simulink model "slproject_f14"  (R2023a)
settings: Solver=VariableStepAuto  StartTime=0.0  StopTime=5  MaxStep=0.1  RelTol=1e-3  EnableMultiTasking=on
undefined symbols (not defined in the file): g, Uo
libraries: wind_gust_lib x1
settings Model: DataDictionary=system_model.sldd  EnableAccessToBaseWorkspace=off  ModifiedByFormat=The MathWorks Inc.  Creator=The MathWorks, Inc.  LastModifiedBy=The MathWorks Inc.
settings SolverCC: AlgebraicLoopSolver=TrustRegion
settings DataIOCC: LimitDataPoints=on  SaveFormat=Array  SaveOutput=off  SignalLogging=off  SaveTime=off  ReturnWorkspaceOutputs=off  SignalLoggingName=slproject_f14
settings OptimizationCC: ExpressionDepthLimit=2147483647  InitFltsAndDblsToZero=on  LifeSpan=inf
settings DebuggingCC: SaveWithParameterizedLinksMsg=none  UnderspecifiedInitializationDetection=Classic  MergeDetectMultiDrivingBlocksExec=none  SignalResolutionControl=TryResolveAllWithWarning  SolverPrmCheckMsg=warning  MultiTaskDSMMsg=warning  MultiTaskCondExecSysMsg=none  FcnCallInpInsideContextMsg=warning  UnconnectedInputMsg=warning  UnconnectedOutputMsg=warning  UnconnectedLineMsg=warning  AllowSymbolicDim=off  StateNameClashWarn=warning  SFUnexpectedBacktrackingDiag=warning  SFNoUnconditionalDefaultTransitionDiag=warning  SFExecutionAtInitializationDiag=none  ArithmeticOperatorsInVariantConditions=warning
settings HardwareCC: ProdBitPerPointer=32  ProdLargestAtomicFloat=None  ProdIntDivRoundTo=Undefined  ProdEndianess=Unspecified  ProdWordSize=32  ProdHWDeviceType=32-bit Generic
settings ModelReferenceCC: EnableRefExpFcnMdlSchedulingChecks=on  ModelReferenceMinAlgLoopOccurrences=on  PropagateSignalLabelsOutOfModel=off
settings SFSimCC: SimUseLocalCustomCode=off  CustomCodeUndefinedFunction=UseInterfaceOnly
settings RTWCC: RTWUseLocalCustomCode=off
settings CodeAppCC: StateflowObjectComments=on
settings GRTTargetCC: TargetFcnLib=ansi_tfl_tmw.mat  TargetLangStandard=C89/C90 (ANSI)  CombineOutputUpdateFcns=off  GRTInterface=on
settings ConfigComp: CovMetricSettings=dw  CovSaveCumulativeToWorkspaceVar=on  CovSaveSingleToWorkspaceVar=on  CovExternalEMLEnable=off  CovSFcnEnable=off

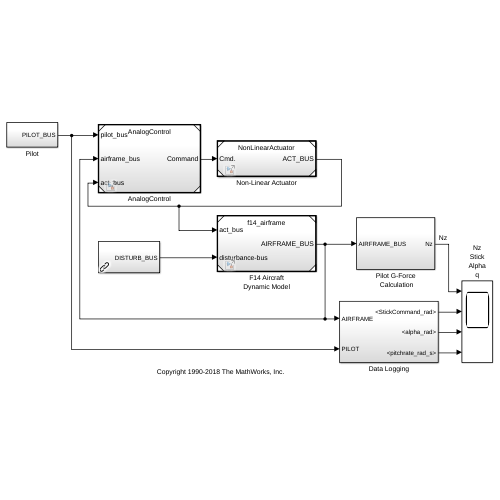
[thumbnail: Simulink's stored preview of the top-level diagram]
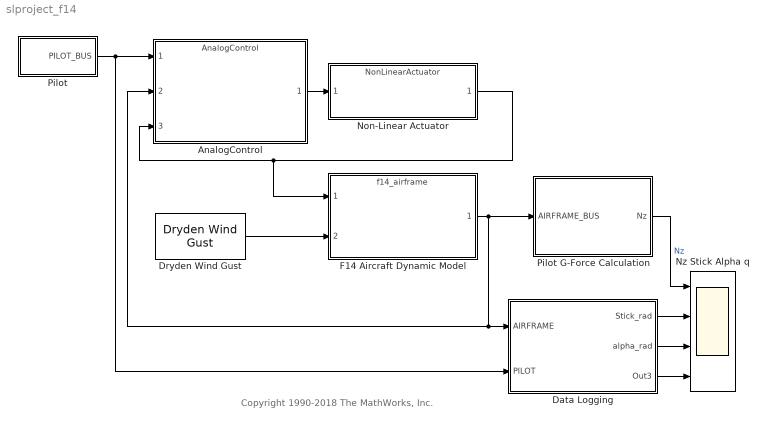
== system slproject_f14 ==
  note: Copyright 1990-2018 The MathWorks, Inc.
  AnalogControl : ModelReference  ModelNameDialog=AnalogControl  SimulationMode=Normal  ModelReferenceVersion=6.0
  Data Logging : Subsystem
  Dryden Wind Gust : wind_gust_lib/Dryden Wind Gust  SystemSampleTime=-1  VariantActivationTime=update diagram  Latency=0  AutoFrameSizeCalculation=off
  F14 Aircraft Dynamic Model : ModelReference  ModelNameDialog=f14_airframe  SimulationMode=Normal  ModelReferenceVersion=9.0
  Non-Linear Actuator : ModelReference  ModelNameDialog=NonLinearActuator  SimulationMode=Normal  ModelReferenceVersion=6.0
  Nz Stick Alpha q : Scope  NumInputPorts=4
  Pilot : Subsystem
  Pilot G-Force Calculation : Subsystem
  wires:
  Pilot/1(PILOT_BUS) -> Data Logging/2(PILOT), AnalogControl/1
  F14 Aircraft Dynamic Model/1 -> Pilot G-Force Calculation/1(AIRFRAME_BUS), AnalogControl/2, Data Logging/1(AIRFRAME)
  Dryden Wind Gust/1 -> F14 Aircraft Dynamic Model/2
  Pilot G-Force Calculation/1(Nz) -> Nz Stick Alpha q/1  "Nz"
  Data Logging/1(Stick_rad) -> Nz Stick Alpha q/2
  Data Logging/2(alpha_rad) -> Nz Stick Alpha q/3
  Data Logging/3(Out3) -> Nz Stick Alpha q/4
  AnalogControl/1 -> Non-Linear Actuator/1
  Non-Linear Actuator/1 -> AnalogControl/3, F14 Aircraft Dynamic Model/1

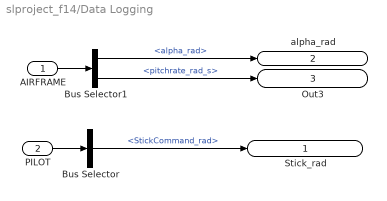
== system slproject_f14/Data Logging ==
  AIRFRAME : Inport
  PILOT : Inport  Port=2
  Bus Selector : BusSelector  OutputSignals=StickCommand_rad
  Bus Selector1 : BusSelector  OutputSignals=alpha_rad,pitchrate_rad_s
  Stick_rad : Outport  VectorParamsAs1DForOutWhenUnconnected=off
  alpha_rad : Outport  Port=2  VectorParamsAs1DForOutWhenUnconnected=off
  Out3 : Outport  Port=3  VectorParamsAs1DForOutWhenUnconnected=off
  wires:
  PILOT/1 -> Bus Selector/1
  AIRFRAME/1 -> Bus Selector1/1
  Bus Selector/1 -> Stick_rad/1  "<StickCommand_rad>"
  Bus Selector1/1 -> alpha_rad/1  "<alpha_rad>"
  Bus Selector1/2 -> Out3/1  "<pitchrate_rad_s>"

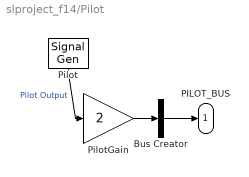
== system slproject_f14/Pilot ==
  Bus Creator : BusCreator  Inputs=1  OutDataTypeStr=Bus: PILOT_BUS
  Pilot : SignalGenerator  WaveForm=square  Frequency=.1
  PilotGain : Gain  Gain=2
  PILOT_BUS : Outport  OutDataTypeStr=Bus: PILOT_BUS  VectorParamsAs1DForOutWhenUnconnected=off
  wires:
  Bus Creator/1 -> PILOT_BUS/1
  PilotGain/1 -> Bus Creator/1
  Pilot/1 -> PilotGain/1  "Pilot Output"

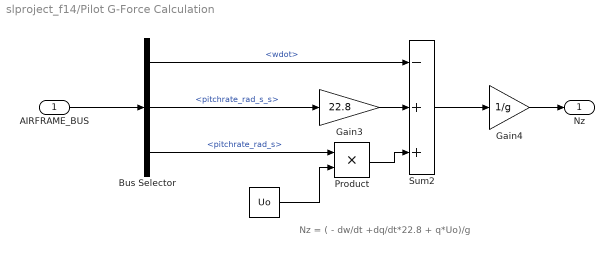
== system slproject_f14/Pilot G-Force Calculation ==
  note: Nz = ( - dw/dt +dq/dt*22.8 + q*Uo)/g
  AIRFRAME_BUS : Inport
  " " : Constant  Value=Uo
  Bus Selector : BusSelector  OutputSignals=wdot,pitchrate_rad_s_s,pitchrate_rad_s
  Gain3 : Gain  Gain=22.8  SaturateOnIntegerOverflow=on  OutDataTypeStr=Inherit: Same as input  ParamDataTypeStr=Inherit: Same as input
  Gain4 : Gain  Gain=1/g  SaturateOnIntegerOverflow=on  OutDataTypeStr=Inherit: Same as input  ParamDataTypeStr=Inherit: Same as input
  Product : Product  InputSameDT=on  RndMeth=Zero  SaturateOnIntegerOverflow=on  OutDataTypeStr=Inherit: Same as first input
  Sum2 : Sum  Inputs=-++  InputSameDT=on  SaturateOnIntegerOverflow=on  OutDataTypeStr=Inherit: Same as first input
  Nz : Outport  VectorParamsAs1DForOutWhenUnconnected=off
  wires:
  " "/1 -> Product/2
  Bus Selector/3 -> Product/1  "<pitchrate_rad_s>"
  Product/1 -> Sum2/3
  Gain3/1 -> Sum2/2
  Bus Selector/2 -> Gain3/1  "<pitchrate_rad_s_s>"
  Gain4/1 -> Nz/1
  Bus Selector/1 -> Sum2/1  "<wdot>"
  Sum2/1 -> Gain4/1
  AIRFRAME_BUS/1 -> Bus Selector/1
